simulink model "Nmpc_pathctl_casadi"  (R2022b)
settings: Solver=FixedStepAuto  StartTime=0.0  StopTime=433  FixedStep=.001  MaxStep=0.01  RelTol=1e-3
values from neighbouring files (symbols this model uses):
  xuanze = Input(15)    [NMPC_casadi_yhn.m]    (also in plotfig.m = 0)
libraries: Solver_SF x1
(part 3 of 11)

== matlab function Nmpc_pathctl_casadi/MATLAB Function2 ==
  data: u input; y output
function y = fcn(u)

y = (u+10);
if y>2000
    y = 2000;
end

== matlab function Nmpc_pathctl_casadi/Burckhardt轮胎侧向力_低附 ==
  data: delta input; Tc_fl input; Tc_fr input; Tc_rl input; Tc_rr input; vx output; vy output; gamma output; vx input; vy input; gamma input; w_fl input; w_fr input; w_rl input; w_rr input; Fy_fl output; Fy_fr output; Fy_rl output; Fy_rr output; fyfl_carsim input; fyfr_carsim input; fyrl_carsim input; fyrr_carsim input; fxfl_carsim input; fxfr_carsim input; fxrl_carsim input; fxrr_carsim input; ax_carsim input
function [vx, vy, gamma, Fy_fl,Fy_fr,Fy_rl,Fy_rr]  = tire_lateral_force(delta, Tc_fl, Tc_fr, Tc_rl, Tc_rr,vx,vy,gamma,w_fl,w_fr,w_rl,w_rr,fyfl_carsim,fyfr_carsim,fyrl_carsim,fyrr_carsim,fxfl_carsim,fxfr_carsim,fxrl_carsim,fxrr_carsim,ax_carsim)

%% 初始化
% vy = 0;%侧向速度
% vx = 0;%纵向速度

% gamma = 0;%横摆角速度
% w_fl = 0;%轮速fl

% w_fr = 0;%轮速fr
% w_rl = 0;%轮速rl
% w_rr = 0;%轮速rr
% Fy_fl = fyfl_carsim;
% Fy_fr = fyfr_carsim;
% Fy_rl = fyrl_carsim;
% Fy_rr = fyrr_carsim;
% Fx_fl = fxfl_carsim;
% Fx_fr = fxfr_carsim;
% Fx_rl = fxrl_carsim;
% Fx_rr = fxrr_carsim;




d = 1.55; %左右轮距
Lf = 1.05;%质心到前轴的距离
Lr = 1.61;%质心到后轴的距离
hcg = 0.54;%质心高度
Iz = 2059.2;%转动惯量
m = 1430;%质量
Iw = 16.8;%车轮转动惯量
Re = 0.3018;%轮胎自由半径
g = 9.8;%重力系数
K_air = 0.9;%空气阻力系数
A = 2.2;%迎风面积
rho_air = 1.206;%空气密度
K_roll = 0.002;%滚动阻力系数
ax = 0;%纵向加速度
ay = 0;%侧向加速度
% c1f = 1.18;%前轮参数
% c1r = 1.49;%后轮参数
% c2f = 10.56;%前轮参数
% c2r = 15.026;%后轮参数
c1f = 1.68;%前轮参数
c1r = 1.49;%后轮参数
c2f = 10.56;%前轮参数
c2r = 15.026;%后轮参数
T = 0.02;%时间步长
c3f = 0.02;
c3r = 0.02;
%% 求解轮胎侧偏角
alpha_fl = - (delta - atan((vy + Lf*gamma)/(vx + gamma*d/2)));
alpha_fr = - (delta - atan((vy + Lf*gamma)/(vx - gamma*d/2)));
alpha_rl = atan((vy - Lr*gamma)/(vx + gamma*d/2));
alpha_rr = atan((vy - Lr*gamma)/(vx - gamma*d/2));
%% 求解滑移率
vx_FL=(vx-1.55/2*gamma)*cos(delta)+(vy+1.05*gamma)*sin(delta);% 车轮fl旋转中心的速度
vx_FR=(vx+1.55/2*gamma)*cos(delta)+(vy+1.05*gamma)*sin(delta);% 车轮fr旋转中心的速度
vx_RL=(vx-1.55/2*gamma);% 车轮rl旋转中心的速度
vx_RR=(vx+1.55/2*gamma);% 车轮rr旋转中心的速度
lambda_fl = (w_fl - vx_FL)/max(vx_FL, w_fl);%滑移率fl计算
lambda_fr = (w_fr - vx_FR)/max(vx_FR, w_fr);%滑移率fr计算
lambda_rl = (w_rl - vx_RL)/max(vx_RL, w_rl);%滑移率rl计算
lambda_rr = (w_rr - vx_RR)/max(vx_RR, w_rr);%滑移率rr计算
% lambda_fl = -1;%滑移率fl计算
% lambda_fr = -1;%滑移率fr计算
% lambda_rl = -1;%滑移率rl计算
% lambda_rr = -1;%滑移率rr计算
%% 垂向载荷计算
Fz_fl = m *(Lr*g/(Lf+Lr)-hcg*ax/(Lf+Lr))* (1/2 );%+320 
Fz_fr = m *(Lr*g/(Lf+Lr)-hcg*ax/(Lf+Lr))* (1/2 );%+320
Fz_rl = m *(Lf*g/(Lf+Lr)-hcg*ax/(Lf+Lr))* (1/2 );%+350
Fz_rr = m *(Lf*g/(Lf+Lr)-hcg*ax/(Lf+Lr))* (1/2 );%+350
%% 轮胎力前轴侧向力计算fyf
s_res_FL = sqrt(lambda_fl.^2 + tan(-alpha_fl).^2);
Ft_FL = Fz_fl * c1f * (1-exp(-c2f*s_res_FL)) - c3f.*s_res_FL;
Fy_fl = 0.9*(-alpha_fl)./s_res_FL.*Ft_FL;%前左轴轮胎侧向力

s_res_FR = sqrt(lambda_fr.^2 + tan(-alpha_fr).^2);
Ft_FR = Fz_fr .* c1f .* (1-exp(-c2f.*s_res_FR)) - c3f.*s_res_FR;
Fy_fr = 0.9*(-alpha_fr)./s_res_FR.*Ft_FR;%前右轮胎侧向力

Fy_F = (0.9*(-alpha_fl)./s_res_FL.*Ft_FL) + (0.9.*(-alpha_fr)./s_res_FR.*Ft_FR);%前轴轮胎侧向力合力
%% 轮胎力后轴侧向力计算fyr
s_res_RL = sqrt(lambda_rl.^2 + tan(-alpha_rl).^2);
Ft_RL = Fz_rl .* c1r.* (1-exp(-c2r.*s_res_RL)) - c3r.*s_res_RL;
Fy_rl = 0.9*(-alpha_rl)./s_res_RL.*Ft_RL;%后左轴轮胎侧向力

s_res_RR = sqrt(lambda_rr.^2 + tan(-alpha_rr).^2);
Ft_RR = Fz_rr .* c1r .* (1-exp(-c2r.*s_res_RR)) - c3r.*s_res_RR;
Fy_rr = 0.9*(-alpha_rr)./s_res_RR.*Ft_RR;%后右轴轮胎侧向力

Fy_R = (0.9*(-alpha_rl)./s_res_RL.*Ft_RL) + (0.9.*(-alpha_rr)./s_res_RR.*Ft_RR);%后轴轮胎侧向力合力

% Fx_fl = Tc_fl/Re;
% Fx_fr = Tc_fr/Re;
% Fx_rl = Tc_rl/Re;
% Fx_rr = Tc_rr/Re;
% 空气阻力计算公式
F_air = 1/2*(A*rho_air*(vx^2))*K_air;
% 滚动阻力系数
F_roll = m*g*K_roll;
% 轮速加速度计算公式
% dot_w_fl=(-Fx_fl*Re+Tc_fl-F_roll*Re)/Iw;
% dot_w_fr=(-Fx_fr*Re+Tc_fr-F_roll*Re)/Iw;
% dot_w_rl=(-Fx_rl*Re+Tc_rl-F_roll*Re)/Iw;
% dot_w_rr=(-Fx_rr*Re+Tc_rr-F_roll*Re)/Iw;

%% 横摆角加速度计算公式
Fy_f = Fy_fl+Fy_fr;
Fy_r = Fy_rl+Fy_rr;
dot_gamma = 1/Iz  *( Fy_f*cos(delta)*Lf - Fy_r*Lr + (Fy_fl - Fy_fr)*sin(delta)*d/2);
gamma = gamma+dot_gamma*T;%进行积分
%% 侧向加速度计算公式
Fy_f = Fy_fl+Fy_fr;
Fy_r = Fy_rl+Fy_rr;
Ay = (Fy_f*cos(delta) + Fy_r )/m;
ay = Ay-gamma*vx;
% vy = vy+ay*T;%进行积分
%% 纵向加速度计算公式
Fy_f = Fy_fl + Fy_fr;
dot_vx = ax_carsim + vy*gamma; 

vx = vx+dot_vx*T;%进行积分
vy = vy+ay*T;%进行积分
